simulink model "MMC_indc"  (R2026a)
settings: Solver=VariableStepAuto  StopTime=10
model workspace (MAT data in the model file):
  L_arm = 40
  L_arm_pow_rat = 14.4
  L_arm_res = 0.4
  L_arm_satcurrent = 7
  L_tolr = 15
  N = 8
  Rarm = 1
  Vdc = 375.5
libraries: nesl_utility x155, fl_lib x111, ee_lib x107
(part 14 of 14)

== matlab function MMC_indc/MATLAB Function2 ==
  data: Gate1u output; Gate2u output; Gate1l output; Gate2l output; vcu input; Su output; vcl input; nu input; nl input; i_upper input; i_lower input; Su_prev input; Sl_prev input; N input; Sl output
function [Gate1u, Gate2u, Gate1l, Gate2l, Su, Sl] = Voltage_Sorting( ...
    vcu, vcl, nu, nl, i_upper, i_lower, Su_prev, Sl_prev, N) %#codegen
%VOLTAGE_SORTING  Sort-and-select balancing for one MMC phase leg, N=8
% half-bridge submodules per arm. Outputs the two
% complementary gate signals each half-bridge SM physically requires.
%
% INPUTS
%   vcu, vcl        - [1xN] upper/lower arm submodule capacitor voltages [V]
%   nu, nl          - required insertion counts
%   i_upper,i_lower - measured arm currents (sign decides charge/discharge)
%   Su_prev,Sl_prev - [1xN] previous cycle's insertion states (hysteresis
%                     input, fed back externally via Unit Delay)
%   N               - submodules per arm (compile-time constant, = 8)
%
% OUTPUTS
%   Gate1u,Gate2u   - [1xN] upper arm gate pairs (Gate2 = NOT(Gate1))
%   Gate1l,Gate2l   - [1xN] lower arm gate pairs
%   Su, Sl          - [1xN] insertion states this cycle (1=insert,0=bypass) --
%                     feed back externally via Unit Delay as next cycle's
%                     Su_prev/Sl_prev

I_DEADBAND = 0.05;  % A -- tune to sensor noise floor at this current scale
V_TOL      = 0.005; % V -- "effectively tied" voltage tolerance at Vc_nom~5V

Su = select_one_arm(vcu, nu, i_upper, Su_prev, N, I_DEADBAND, V_TOL);
Sl = select_one_arm(vcl, nl, i_lower, Sl_prev, N, I_DEADBAND, V_TOL);

Gate1u = Su;              Gate2u = double(~Su);
Gate1l = Sl;              Gate2l = double(~Sl);
end

function S = select_one_arm(vc, n_ins, i_arm, S_prev, N, I_DEADBAND, V_TOL)
S = zeros(1,N);
[~, idx_ascend] = sort(vc, 'ascend');   % idx_ascend(1) = lowest-voltage SM

if i_arm > I_DEADBAND
    idx_sel = idx_ascend;                 % charging: lowest-V first
elseif i_arm < -I_DEADBAND
    idx_sel = idx_ascend(N:-1:1);          % discharging: highest-V first
else
    % Deadband: pick whichever direction needs fewer state changes,
    % avoiding chatter when i_arm sits near zero (noise-driven flips).
    cand_charge    = zeros(1,N); cand_charge(idx_ascend(1:n_ins)) = 1;
    cand_discharge = zeros(1,N); cand_discharge(idx_ascend(N-n_ins+1:N)) = 1;
    if sum(abs(cand_charge - S_prev)) <= sum(abs(cand_discharge - S_prev))
        idx_sel = idx_ascend;
    else
        idx_sel = idx_ascend(N:-1:1);
    end
end

S(idx_sel(1:n_ins)) = 1;

% Hysteresis pass: near-tied SMs swap back to the previous cycle's
% assignment -- physically equivalent output, one fewer commutation.
for j = 1:N
    if S(j) ~= S_prev(j)
        for k = 1:N
            if k ~= j && S(k)==S_prev(j) && S_prev(k)==S(j) ...
                    && abs(vc(j)-vc(k)) < V_TOL
                tmp = S(j); S(j) = S(k); S(k) = tmp;
            end
        end
    end
end
end
